simulink model "balance_robot_chuanlian"  (R2024a)
settings: Solver=VariableStepAuto  StartTime=0.0  StopTime=10.0  RelTol=1e-3
values from neighbouring files (symbols this model uses):
  X = [x1, x2, x1sq, x2sq, x1x2]    [k_calc.m]
undefined symbols (not defined in the file or in its folder): Y, Z
libraries: sm_lib x114, nesl_utility x1
(part 1 of 2)
settings Model: Creator=zhuho  LastModifiedBy=zhuho

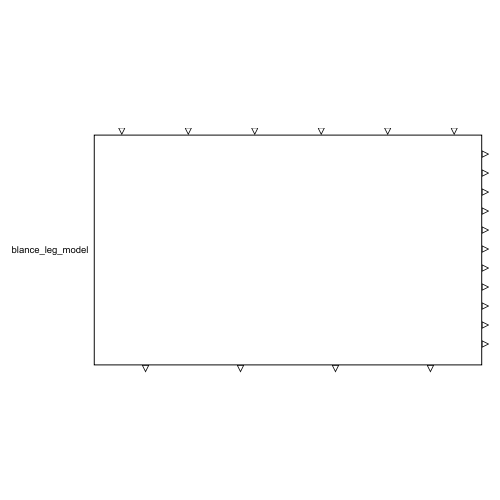
[thumbnail: Simulink's stored preview of the top-level diagram]
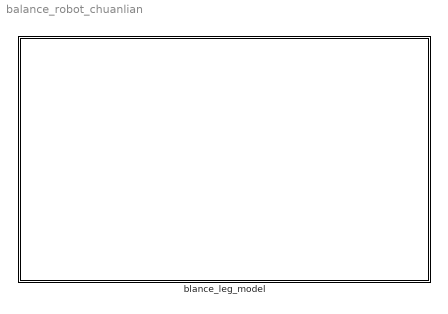
== system balance_robot_chuanlian ==
  blance_leg_model : Subsystem
      settings: PortSchema="{\"entries\":[{\"content\":{\"sides\":[{\"content\":{\"connectorIds\":[\"LConn1\",\"LConn2\",\"LConn3\",\"LConn4\",\"LConn5\",\"LConn6\"]},\"type\":\"ConnectorPlacement.EquallySpacedRectSide\",\"uuid\":\"ed635f35-0836-4900-93e3-56fc3520c8de\"},{\"content\":{\"connectorIds\":[\"RConn1\",\"RConn2\",\"RConn3\",\"RConn4\"],\"side\":\"RIGHT\"},\"type\":\"ConnectorPlacement.EquallySpacedRectSide\",\"uuid\":\"bb235ec0-defd-4ad9-96f6-8533dab3fbd9\"},{\"content\":{\"side\":\"TOP\"},\"type\":\"ConnectorPlacement.EquallySpacedRectSide\",\"uuid\":\"d719db37-8b3a-4344-b330-944fde418334\"},{\"content\":{\"connectorIds\":[\"RConn5\",\"RConn6\",\"RConn7\",\"RConn8\",\"RConn9\",\"RConn10\",\"RConn11\",\"RConn12\",\"RConn13\",\"RConn14\",\"RConn15\"],\"side\":\"BOTTOM\"},\"type\":\"ConnectorPlacement.EquallySpacedRectSide\",\"uuid\":\"20f9270b-6ab1-4e89-bf00-e838d12c3c13\"}]},\"type\":\"ConnectorPlacement.EquallySpacedConnector\",\"uuid\":\"a2f25b71-0047-4a2d-a238-dad76f034ab1\"}],\"packageUris\":[\"http://schema.mathworks.com/mf0/Connector/R2020b\"],\"version\":\"1.0\"}"
